simulink model "sim_sil_top_s32k1xx"  (Simulink 9.0)
settings: Solver=FixedStepDiscrete  StartTime=0.0  StopTime=100.0  FixedStep=0.01  RelTol=1e-3  EnableMultiTasking=on
InitFcn:
  | mbd_s32k_consistency_checks(bdroot(gcs));
settings Model: Creator=NXP MBDT Team  LastModifiedBy=nxf35172
settings DataIOCC: LimitDataPoints=on
settings OptimizationCC: DefaultParameterBehavior=Inlined  EnhancedBackFolding=on  PassReuseOutputArgsAs=Individual arguments  LifeSpan=auto  OptimizeBlockOrder=speed  DifferentSizesBufferReuse=on
settings DebuggingCC: UnderspecifiedInitializationDetection=Simplified  MergeDetectMultiDrivingBlocksExec=error  SolverPrmCheckMsg=warning  InheritedTsInSrcMsg=none  ParameterTunabilityLossMsg=error  AllowSymbolicDim=off
settings HardwareCC: ProdIntDivRoundTo=Zero  ProdEndianess=LittleEndian  ProdHWDeviceType=Generic->Custom
settings SFSimCC: MATLABDynamicMemAlloc=off
settings RTWCC: SystemTargetFile=mbd_s32k.tlc  MakeCommand=mbd_s32k_make_rtw COPY_MDLREF_INCLUDES=0  TemplateMakefile=mbd_s32k.tmf  Description=Model Based Design Toolbox S32K1xx Code Generation Target  GenerateReport=on  IncludeHyperlinkInReport=on  LaunchReport=on  PortableWordSizes=on  CreateSILPILBlock=PIL  GenerateTraceInfo=on  GenerateTraceReport=on  GenerateTraceReportSl=on  GenerateTraceReportSf=on  GenerateTraceReportEml=on
settings CodeAppCC: ForceParamTrailComments=on  IgnoreCustomStorageClasses=off  MaxIdLength=63  OperatorAnnotations=on  SimulinkDataObjDesc=on  SFDataObjDesc=on  InsertBlockDesc=on  StateflowObjectComments=off
settings STFCustomTargetCC: MultiwordLength=256  GenerateSampleERTMain=on  CombineOutputUpdateFcns=on  SuppressErrorStatus=on  ERTCustomFileBanners=on  SupportAbsoluteTime=off  SupportContinuousTime=off  SupportNonInlinedSFcns=off  RemoveResetFunc=on  MATLABClassNameForMDSCustomization=Simulink.SoftwareTarget.ERTCustomization  GRTInterface=off  SystemTargetFile=mbd_s32k.tlc
settings ERTTargetCC: GenerateSampleERTMain=on  ParMdlRefBuildCompliant=off  CompOptLevelCompliant=off  ConcurrentExecutionCompliant=off  SuppressErrorStatus=on  SupportAbsoluteTime=off  ModelStepFunctionPrototypeControlCompliant=off  CPPClassGenCompliant=off  UseToolchainInfoCompliant=off  InlinedParameterPlacement=NonHierarchical  ERTCustomFileTemplate=example_file_process.tlc

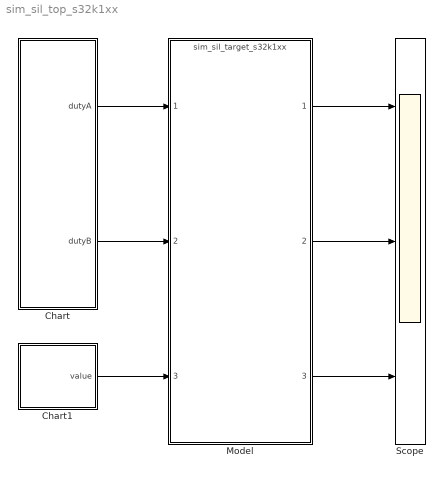
== system sim_sil_top_s32k1xx ==
  Chart : Stateflow chart  TreatAsAtomicUnit=on
  Chart1 : Stateflow chart  TreatAsAtomicUnit=on
  Model : ModelReference  ModelNameDialog=sim_sil_target_s32k1xx.mdl  SimulationMode=Software-in-the-loop (SIL)  ModelReferenceVersion=1.101
  Scope : Scope  NumInputPorts=3
  wires:
  Chart/1(dutyA) -> Model/1
  Chart/2(dutyB) -> Model/2
  Chart1/1(value) -> Model/3
  Model/1 -> Scope/1
  Model/2 -> Scope/2
  Model/3 -> Scope/3

== stateflow chart Chart ==
  settings: executeAtInitialization=1
  state A
    du:
    dutyA=0.75;
    dutyB=0.15;
    cntr=cntr+1;
  state A1
    du:
    dutyA=0.0;
    dutyB=0.85;
    cntr=cntr-1;
  (default) -> A : {cntr=0;}
  A1 -> A : [cntr < 2]
  A -> A1 : [cntr > 50]
  data: cntr local uint32 =0; dutyA output single [0..100]; dutyB output single [0..100]

== stateflow chart Chart1 ==
  settings: executeAtInitialization=1
  state A
    du:
    cntr=cntr+100;
    value=cntr;
    ex:
    cntr = -32700;
  (default) -> A : {cntr=0;}
  A -> A : [cntr >= 32700]
  data: cntr local single =0; value output int16
